simulink model "modele_ballon"  (Simulink 9.1)
settings: Solver=VariableStepAuto  StartTime=0.0  StopTime=100  MaxStep=0.01  RelTol=1e-4  EnableMultiTasking=on
settings Model: SuppressorTable=22 serialization::archive 11 0 6 0 0 0 1 0  Creator=krauthl  LastModifiedBy=krauthl
settings DataIOCC: LimitDataPoints=on  SaveFormat=Dataset  SaveOutput=off  SaveTime=off
settings OptimizationCC: ExpressionDepthLimit=2147483647  LifeSpan=1
settings DebuggingCC: FcnCallInpInsideContextMsg=warning  AllowSymbolicDim=off  StateNameClashWarn=warning
settings HardwareCC: ProdBitPerPointer=64  ProdBitPerSizeT=64  ProdBitPerPtrDiffT=64  ProdLargestAtomicFloat=Float  ProdIntDivRoundTo=Zero  ProdEndianess=LittleEndian  ProdWordSize=64  ProdHWDeviceType=Intel->x86-64 (Windows64)
settings ModelReferenceCC: PropagateSignalLabelsOutOfModel=on
settings GRTTargetCC: GeneratePreprocessorConditionals=Disable all
settings ConfigComp: CovMetricSettings=dwe  CovHtmlReporting=off  CovSaveCumulativeToWorkspaceVar=off  CovSaveSingleToWorkspaceVar=off  CovExternalEMLEnable=on

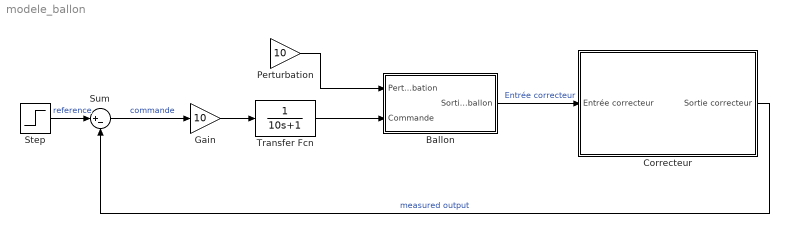
== system modele_ballon ==
  "Ballon " : Subsystem
  "Correcteur " : Subsystem
  Gain : Gain  Gain=10
  "Perturbation " : Gain  Gain=10
  Step : Step  SampleTime=0
  Sum : Sum  Inputs=|+-
  Transfer Fcn : TransferFcn  Denominator=[10 1]
  wires:
  Step/1 -> Sum/1  "reference"
  "Correcteur "/1("Sortie correcteur ") -> Sum/2  "measured output"
  Sum/1 -> Gain/1  "commande"
  "Ballon "/1("Sortie ballon ") -> "Correcteur "/1("Entrée correcteur ")  "Entrée correcteur"
  "Perturbation "/1 -> "Ballon "/1("Perturbation ")
  Transfer Fcn/1 -> "Ballon "/2("Commande ")
  Gain/1 -> Transfer Fcn/1

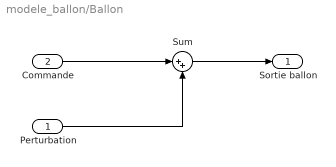
== system modele_ballon/Ballon  ==
  "Perturbation " : Inport
  "Commande " : Inport  Port=2
  Sum : Sum  Inputs=|++
  "Sortie ballon " : Outport
  wires:
  "Commande "/1 -> Sum/1
  Sum/1 -> "Sortie ballon "/1
  "Perturbation "/1 -> Sum/2

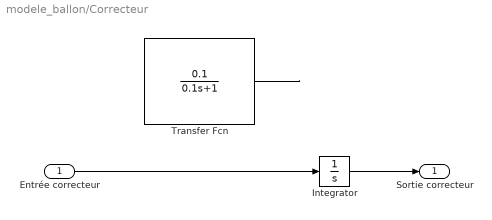
== system modele_ballon/Correcteur  ==
  "Entrée correcteur " : Inport
  Integrator : Integrator
  Transfer Fcn : TransferFcn  Numerator=[0.1]  Denominator=[0.1 1]
  "Sortie correcteur " : Outport
  wires:
  "Entrée correcteur "/1 -> Integrator/1
  Integrator/1 -> "Sortie correcteur "/1
  Transfer Fcn/1 -> ?
